simulink model "CAD_exp2_5"  (R2019a)
settings: Solver=VariableStepAuto  StartTime=0.0  StopTime=40  RelTol=1e-3
settings Model: Creator=83621  LastModifiedBy=83621

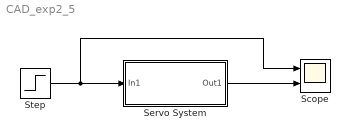
== system CAD_exp2_5 ==
  Scope : Scope  NumInputPorts=2
  Servo System : Subsystem  mask{Kc1=100, Kc2=1}
  Step : Step  SampleTime=0
  wires:
  Step/1 -> Scope/1, Servo System/1(In1)
  Servo System/1(Out1) -> Scope/2

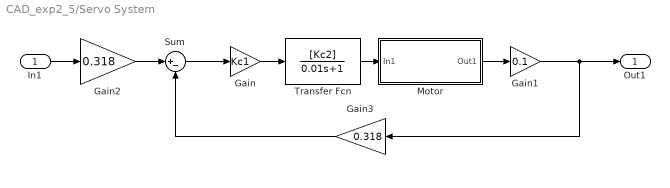
== system CAD_exp2_5/Servo System ==
  In1 : Inport
  Gain : Gain  Gain=Kc1
  Gain1 : Gain  Gain=0.1
  Gain2 : Gain  Gain=0.318
  Gain3 : Gain  Gain=0.318
  Motor : Subsystem
  Sum : Sum  Inputs=|+-
  Transfer Fcn : TransferFcn  Numerator=[Kc2]  Denominator=[0.01 1]
  Out1 : Outport
  wires:
  Gain/1 -> Transfer Fcn/1
  Transfer Fcn/1 -> Motor/1(In1)
  Motor/1(Out1) -> Gain1/1
  In1/1 -> Gain2/1
  Gain2/1 -> Sum/1
  Sum/1 -> Gain/1
  Gain1/1 -> Gain3/1, Out1/1
  Gain3/1 -> Sum/2

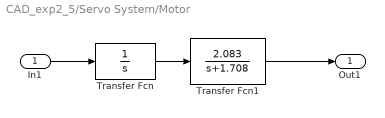
== system CAD_exp2_5/Servo System/Motor ==
  In1 : Inport
  Transfer Fcn : TransferFcn  Denominator=[1 0]
  Transfer Fcn1 : TransferFcn  Numerator=[2.083]  Denominator=[1 1.708]
  Out1 : Outport
  wires:
  Transfer Fcn/1 -> Transfer Fcn1/1
  In1/1 -> Transfer Fcn/1
  Transfer Fcn1/1 -> Out1/1
